simulink model "Transimpedance1"  (R2020b)
settings: Solver=VariableStepAuto  StartTime=0.0  StopTime=10  RelTol=1e-3
libraries: fl_lib x9, nesl_utility x4, ee_lib x3
settings Model: Creator=Miodrag Bolic  LastModifiedBy=bolic

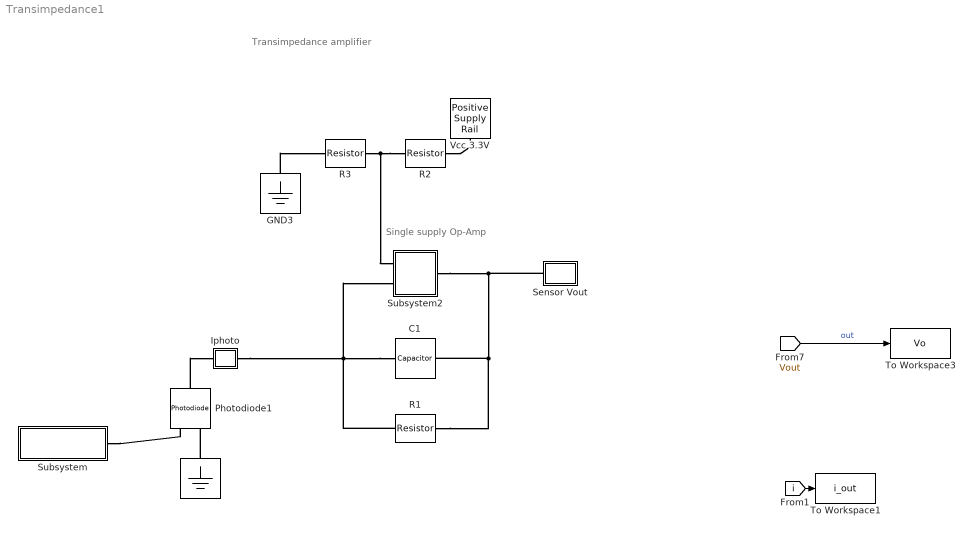
== system Transimpedance1 ==
  note: Single supply
      | Op-Amp
  note: Transimpedance amplifier
  " " : fl_lib/Electrical/Electrical Elements/Electrical Reference
  C1 : fl_lib/Electrical/Electrical Elements/Capacitor  c=5 nF  r=0 Ohm  g=0 1/Ohm  i_specify=off  i_priority=High  i=0 A  i_nominal_specify=off  i_nominal_unit=A  i_nominal_value=1  v_specify=off  v_priority=High  v=0 V  v_nominal_specify=off  v_nominal_unit=V  v_nominal_value=1  vc_specify=off  vc_priority=High  vc=0 V  vc_nominal_specify=off  vc_nominal_unit=V  vc_nominal_value=1
      settings: AttributesFormatString=%<c> %<c_unit>  SourceProductName=Foundation Library
  GND3 : fl_lib/Electrical/Electrical Elements/Electrical Reference
      settings: AttributesFormatString=\n
  Iphoto : Subsystem
      mask Display: disp('i')
  Photodiode1 : ee_lib/Sensors & Transducers/Photodiode  prmFlux=1  Imeas=10 uA  FluxD=10 W/m^2  G=5e-6 m^2*A/W  prmExp=2  I2=0.1 A  V2=1.3 V  IS=5e-9 A  ec=3  RS=0.001 Ohm  Tmeas=25 degC  C_param=1  CJ=70 pF  CJ0=70 pF  VJ=1 V  Mgrad=0.5  Vvec=[ 0.1 10 100 ] V  Cvec=[ 45 30 6 ] pF  FC=0.5  T_param=1  IS_T2=2.5e-7 A  I1_T2=0.07000000000000001 A  V1_T2=1.3 V  Tmeas2=125 degC  EG_param=1  EG=1.11 eV  XTI_param=1  XTI=3  Tdevice=25 degC  i_capacitor_specify=off  i_capacitor_priority=High  i_capacitor=0 A  i_capacitor_nominal_specify=off  i_capacitor_nominal_unit=A  i_capacitor_nominal_value=1  v_capacitor_specify=off  v_capacitor_priority=None  v_capacitor=0 V  v_capacitor_nominal_specify=off  v_capacitor_nominal_unit=V  v_capacitor_nominal_value=1  thermal_network_parameterization=ee.enum.thermalNetworkTopology.cauer  Rth=[0, 10] K/W  Rth_Foster=[4, 6] K/W  thermal_mass_parameterization=ee.enum.thermalNetwork.timeconstant  thermal_mass=[0, 1] J/K  thermal_mass_Foster=[1.5, 3] J/K  thermal_time_constant=[0, 10] s  thermal_time_constant_Foster=[6, 18] s  thermal_mass_initial_temperatures=[25, 25] degC
      settings: SourceProductBaseCode=PS  InternalSimscapePortConfiguration="{\"Bottom\":[],\"Left\":[{\"id\":\"W\",\"label\":\"W\",\"type\":\"input\"},{\"id\":\"p\",\"label\":\"\",\"type\":\"foundation.electrical.electrical\"}],\"Right\":[{\"id\":\"n\",\"label\":\"\",\"type\":\"foundation.electrical.electrical\"}],\"Top\":[]}"
  R1 : fl_lib/Electrical/Electrical Elements/Resistor  R=200 kOhm  i_specify=off  i_priority=High  i=0 A  i_nominal_specify=off  i_nominal_unit=A  i_nominal_value=1  v_specify=off  v_priority=High  v=0 V  v_nominal_specify=off  v_nominal_unit=V  v_nominal_value=1
      settings: AttributesFormatString=%<R> %<R_unit>  SourceProductName=Foundation Library
  R2 : fl_lib/Electrical/Electrical Elements/Resistor  R=10 kOhm  i_specify=off  i_priority=None  i=0 A  i_nominal_specify=off  i_nominal_unit=A  i_nominal_value=1  v_specify=off  v_priority=None  v=0 V  v_nominal_specify=off  v_nominal_unit=V  v_nominal_value=1
      settings: AttributesFormatString=|
      | %<R>
      | %<R_unit>
  R3 : fl_lib/Electrical/Electrical Elements/Resistor  R=1.2 kOhm  i_specify=off  i_priority=None  i=0 A  i_nominal_specify=off  i_nominal_unit=A  i_nominal_value=1  v_specify=off  v_priority=None  v=0 V  v_nominal_specify=off  v_nominal_unit=V  v_nominal_value=1
      settings: AttributesFormatString=%<R> %<R_unit>
  Sensor Vout : Subsystem
      mask Display: disp('Vo')
  Subsystem : Subsystem
      mask Display: disp('Irradiance')
  Subsystem2 : Subsystem
      mask Display: image('op_amp_plus_up.png')
  To Workspace1 : ToWorkspace  VariableName=i_out  SaveFormat=Timeseries  SampleTime=-1
  To Workspace3 : ToWorkspace  VariableName=Vo  SaveFormat=Timeseries  SampleTime=0.001
  Vcc 3.3V : ee_lib/Sources/Positive Supply Rail  v0=3.3 V
      settings: SourceProductBaseCode=PS  InternalSimscapePortConfiguration="{\"Bottom\":[],\"Left\":[],\"Right\":[{\"id\":\"p\",\"label\":\"\",\"type\":\"foundation.electrical.electrical\"}],\"Top\":[]}"
  wires:
  [Vout] -> To Workspace3/1  "out"
  [i] -> To Workspace1/1
  connections:
  Sensor Vout/LConn1 -- R1/RConn1 -- C1/RConn1 -- Subsystem2/RConn1
  R2/RConn1 -- R3/LConn1 -- Subsystem2/LConn1
  C1/LConn1 -- Iphoto/LConn1 -- R1/LConn1 -- Subsystem2/LConn2
  " "/LConn1 -- Photodiode1/LConn2
  GND3/LConn1 -- R3/RConn1
  R2/LConn1 -- Vcc 3.3V/RConn1
  Subsystem/RConn1 -- Photodiode1/LConn1
  Photodiode1/RConn1 -- Iphoto/RConn1

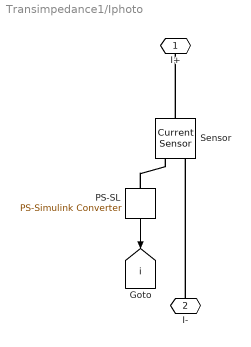
== system Transimpedance1/Iphoto ==
  PS-SL : nesl_utility/PS-Simulink Converter  PhysicalDomain=network_engine_domain  SubClassName=ps_output  LeftPortType=input  RightPortType=output  PseudoPeriodic=off  Frequencies=[]  Unit=1  AffineConversion=off
  Sensor : fl_lib/Electrical/Electrical Sensors/Current Sensor
      settings: SourceProductName=Foundation Library
  I+ : PMIOPort  Side=Right
  I- : PMIOPort  Port=2  Side=Left
  tag scope: i=global
  wires:
  PS-SL/1 -> [i]
  connections:
  PS-SL/LConn1 -- Sensor/RConn1
  Sensor/LConn1 -- I+/RConn1
  I-/RConn1 -- Sensor/RConn2

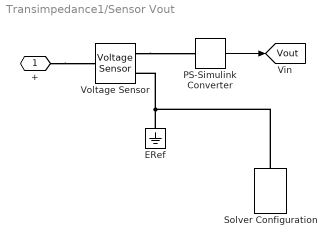
== system Transimpedance1/Sensor Vout ==
  ERef : fl_lib/Electrical/Electrical Elements/Electrical Reference
      settings: SourceProductName=Foundation Library
  PS-Simulink Converter : nesl_utility/PS-Simulink Converter  PhysicalDomain=network_engine_domain  SubClassName=ps_output  LeftPortType=input  RightPortType=output  PseudoPeriodic=off  Frequencies=[]  Unit=1  AffineConversion=off
      settings: SourceProductName=Utilities
  Solver Configuration : nesl_utility/Solver Configuration  PhysicalDomain=network_engine_domain  SubClassName=solver  LeftPortType=input  RightPortType=generic  Tones=[]  Harmonics=[]  SimulateNoise=off  Profile=off  UseLocalSampling=off  EnableSwitchedLinearOptims=on  FrequencyDomain=off  UseCCode=off  RelTol=0.001  AbsTol=1e-06  MinStep=1e-09  ToWorkspace=off  RevertToSquareIcSolve=off  NumHomotopyIterations=100  PhasorMode=off  PhasorModeNumHarmonics=1  DoDC=off  ResidualTolerance=1e-09  UseLocalSolver=off  LocalSolverChoice=NE_TRAPEZOIDAL_ADVANCER  LocalSolverSampleTime=0.0000001  DoFixedCost=off  MaxNonlinIter=3  MaxModeIter=2  ComputeImpulses=off  ImpulseIterations=2  LinearAlgebra=Sparse  EquationFormulation=NE_TIME_EF  DelaysMemoryBudget=1024  AutomaticFiltering=on  FilteringTimeConstant=0.00001  PartitionStorageMethod=AS_NEEDED  PartitionMemoryBudget=1024  PartitionMethod=ROBUST
  Voltage Sensor : fl_lib/Electrical/Electrical Sensors/Voltage Sensor
      settings: SourceProductName=Foundation Library
  + : PMIOPort  Side=Left
  tag scope: Vout=global
  wires:
  PS-Simulink Converter/1 -> [Vout]
  connections:
  ERef/LConn1 -- Solver Configuration/RConn1 -- Voltage Sensor/RConn2
  Voltage Sensor/RConn1 -- PS-Simulink Converter/LConn1
  +/RConn1 -- Voltage Sensor/LConn1

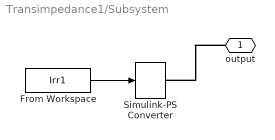
== system Transimpedance1/Subsystem ==
  From Workspace : FromWorkspace  VariableName=Irr1  SampleTime=0.0001  OutputAfterFinalValue=Setting to zero
  Simulink-PS Converter : nesl_utility/Simulink-PS Converter  PhysicalDomain=network_engine_domain  SubClassName=ps_input  LeftPortType=input  RightPortType=output  PseudoPeriodic=off  Frequencies=[]  NoiseDistribution=none  NoiseParameters=[]  Unit=1  AffineConversion=off  FilteringAndDerivatives=zero  SimscapeFilterOrder=1  InputFilterTimeConstant=0.001  UdotUserProvided=1
  output : PMIOPort  Side=Right
  wires:
  From Workspace/1 -> Simulink-PS Converter/1
  connections:
  output/RConn1 -- Simulink-PS Converter/RConn1

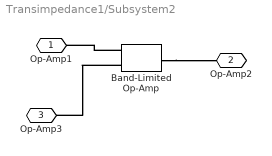
== system Transimpedance1/Subsystem2 ==
  Band-Limited Op-Amp : ee_lib/Integrated Circuits/Band-Limited Op-Amp  A=1000  Rin=1e8 Ohm  Rout=100 Ohm  Vmin=0 V  Vmax=3.3 V  Vdotmax=1000 V/s  f=1e5 Hz  V0=0 V
      settings: SourceProductBaseCode=SN
  Op-Amp1 : PMIOPort  Side=Left
  Op-Amp2 : PMIOPort  Port=2  Side=Right
  Op-Amp3 : PMIOPort  Port=3  Side=Left
  connections:
  Band-Limited Op-Amp/LConn1 -- Op-Amp1/RConn1
  Band-Limited Op-Amp/LConn2 -- Op-Amp3/RConn1
  Band-Limited Op-Amp/RConn1 -- Op-Amp2/RConn1
